simulink model "TVC_6DOF_Model_WJHedits_2024a"  (R2024b)
settings: Solver=VariableStepAuto  StartTime=0.0  StopTime=8  FixedStep=.0001  RelTol=1e-6
values from neighbouring files (symbols this model uses):
  dt = 1/400    (= 0.0025)    [quaternionLQR_WJHedits.m]
  K = lqr(A,B, Q, R)    [quaternionLQR_WJHedits.m]
  mass = .89    (= 0.89)    [quaternionLQR_WJHedits.m]
  maxGimbal = deg2rad(8)    [quaternionLQR_WJHedits.m]
  momentArm = 0.49    [quaternionLQR_WJHedits.m]
  q_init = angle2quat(euler_init(3),euler_init(2),euler_init(1),'ZYX')    [quaternionLQR_WJHedits.m]
  servoRatio = 3.3    [quaternionLQR_WJHedits.m]
  T = 15    [quaternionLQR_WJHedits.m]
  thrust = data{:,2}    [quaternionLQR_WJHedits.m]
  time = data{:,1}    [quaternionLQR_WJHedits.m]
undefined symbols (not defined in the file or in its folder): prop
libraries: simulink x4, sharedtransform x1, shared6dof x1, aerolibanim x1
settings Model: Creator=lucan  LastModifiedBy=C27Nathan.Aldridge

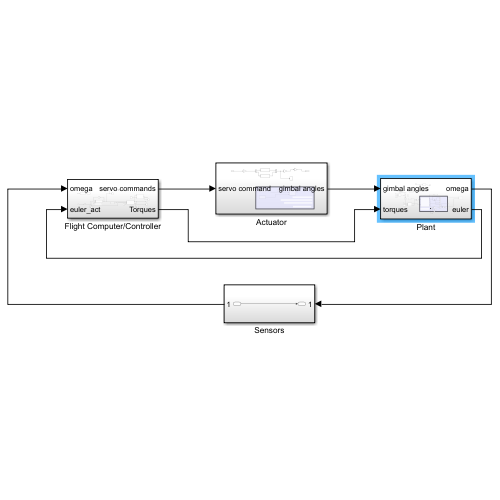
[thumbnail: Simulink's stored preview of the top-level diagram]
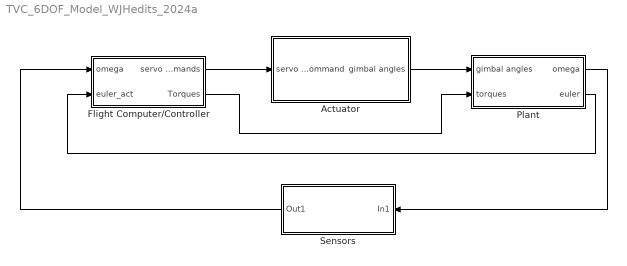
== system TVC_6DOF_Model_WJHedits_2024a ==
  Actuator : Subsystem
  Flight Computer/Controller : Subsystem
  Plant : Subsystem
  Sensors : Subsystem
  wires:
  Plant/1(omega) -> Sensors/1(In1)
  Sensors/1(Out1) -> Flight Computer/Controller/1(omega)
  Flight Computer/Controller/1(" servo commands") -> Actuator/1(servo command)
  Actuator/1(gimbal angles) -> Plant/1(gimbal angles)
  Plant/2(euler) -> Flight Computer/Controller/2(euler_act)
  Flight Computer/Controller/2(Torques) -> Plant/2(torques)

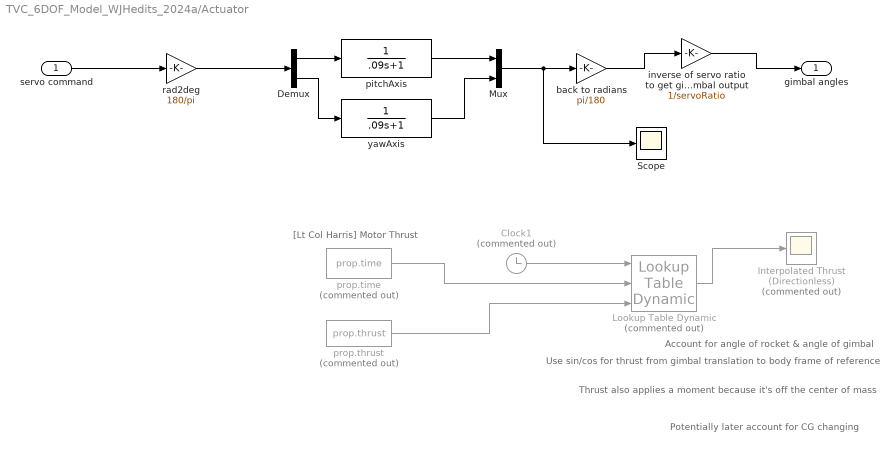
== system TVC_6DOF_Model_WJHedits_2024a/Actuator ==
  note: Potentially later account for CG changing
  note: Thrust also applies a moment because it's off the center of mass
  note: Account for angle of rocket & angle of gimbal
  note: [Lt Col Harris] Motor Thrust
  note: Use sin/cos for thrust from gimbal translation to body frame of reference
  servo command : Inport
  Clock1 : Clock  Commented=on
  Demux : Demux  Outputs=2
  Interpolated Thrust (Directionless) : Scope  Commented=on
  Lookup Table Dynamic : simulink/Lookup Tables/Lookup Table Dynamic  Commented=on  LookUpMeth=Interpolation-Use End Values  OutDataType=fixdt('double')  OutScaling=[]  OutputDataTypeScalingMode=Specify via dialog  OutDataTypeStr=double  DoSatur=off
  Mux : Mux  Inputs=2
  Scope : Scope
  back to radians : Gain  Gain=pi/180
  inverse of servo ratio to get gimbal output : Gain  Gain=1/servoRatio
  pitchAxis : TransferFcn  Denominator=[.09 1]  ContinuousStateAttributes='servoposition'
  prop.thrust : Constant  Commented=on  Value=prop.thrust
  prop.time : Constant  Commented=on  Value=prop.time
  rad2deg : Gain  Gain=180/pi
  yawAxis : TransferFcn  Denominator=[.09 1]  ContinuousStateAttributes='servoposition'
  gimbal angles : Outport
  wires:
  prop.time/1 -> Lookup Table Dynamic/2
  prop.thrust/1 -> Lookup Table Dynamic/3
  Lookup Table Dynamic/1 -> Interpolated Thrust (Directionless)/1
  Clock1/1 -> Lookup Table Dynamic/1
  servo command/1 -> rad2deg/1
  Demux/2 -> yawAxis/1
  Demux/1 -> pitchAxis/1
  pitchAxis/1 -> Mux/1
  yawAxis/1 -> Mux/2
  Mux/1 -> Scope/1, back to radians/1
  inverse of servo ratio to get gimbal output/1 -> gimbal angles/1
  rad2deg/1 -> Demux/1
  back to radians/1 -> inverse of servo ratio to get gimbal output/1

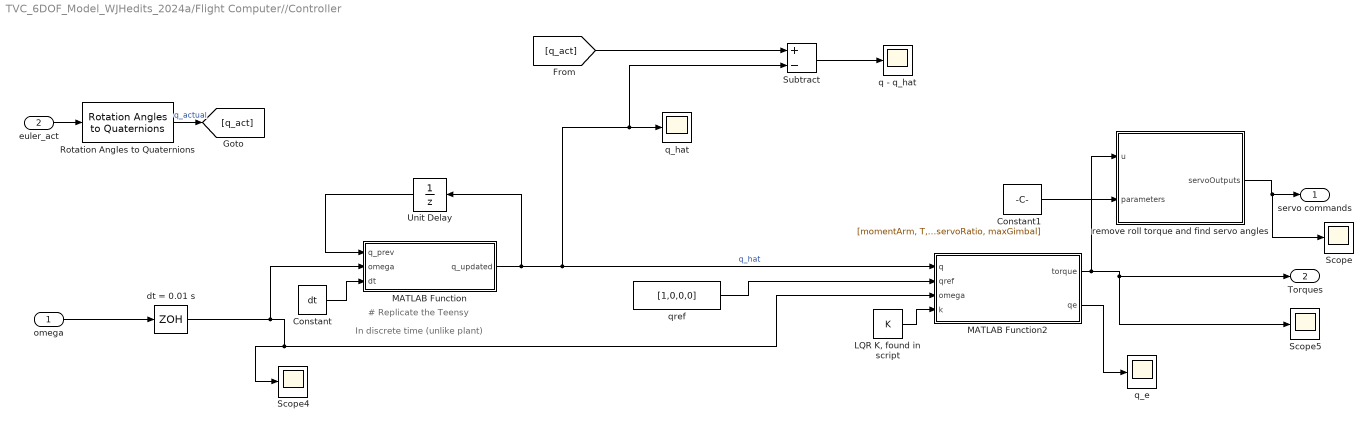
== system TVC_6DOF_Model_WJHedits_2024a/Flight Computer//Controller ==
  note: In discrete time (unlike plant)
  note: # Replicate the Teensy
  omega : Inport
  euler_act : Inport  Port=2
  Constant : Constant  Value=dt
  Constant1 : Constant  Value=[momentArm, T, servoRatio, maxGimbal]
  "LQR K, found in script" : Constant  Value=K
  MATLAB Function : MATLAB Function  TreatAsAtomicUnit=on
  MATLAB Function2 : MATLAB Function  TreatAsAtomicUnit=on
  Rotation Angles to Quaternions : sharedtransform/Rotation Angles to Quaternions  rotationOrder=XYZ  aMode=aMode
  Scope : Scope
  Scope4 : Scope
  Scope5 : Scope
  Subtract : Sum  Inputs=+-
  Unit Delay : UnitDelay  InitialCondition=q_init  SampleTime=-1  HasFrameUpgradeWarning=on
  dt = 0.01 s : ZeroOrderHold  SampleTime=dt
  q - q_hat : Scope
  q_e : Scope
  q_hat : Scope
  qref : Constant  Value=[1,0,0,0]
  remove roll torque and find servo angles : MATLAB Function  TreatAsAtomicUnit=on
  " servo commands" : Outport
  Torques : Outport  Port=2
  wires:
  Constant/1 -> MATLAB Function/3(dt)
  "LQR K, found in script"/1 -> MATLAB Function2/4(k)
  qref/1 -> MATLAB Function2/2(qref)
  MATLAB Function2/2(qe) -> q_e/1
  euler_act/1 -> Rotation Angles to Quaternions/1
  MATLAB Function/1(q_updated) -> MATLAB Function2/1(q), Subtract/2, q_hat/1, Unit Delay/1  "q_hat"
  MATLAB Function2/1(torque) -> Torques/1, Scope5/1, remove roll torque and find servo angles/1(u)
  omega/1 -> dt = 0.01 s/1
  remove roll torque and find servo angles/1(servoOutputs) -> Scope/1, " servo commands"/1
  Unit Delay/1 -> MATLAB Function/1(q_prev)
  Subtract/1 -> q - q_hat/1
  Rotation Angles to Quaternions/1 -> [q_act]  "q_actual"
  [q_act] -> Subtract/1
  dt = 0.01 s/1 -> Scope4/1, MATLAB Function2/3(omega), MATLAB Function/2(omega)
  Constant1/1 -> remove roll torque and find servo angles/2(parameters)

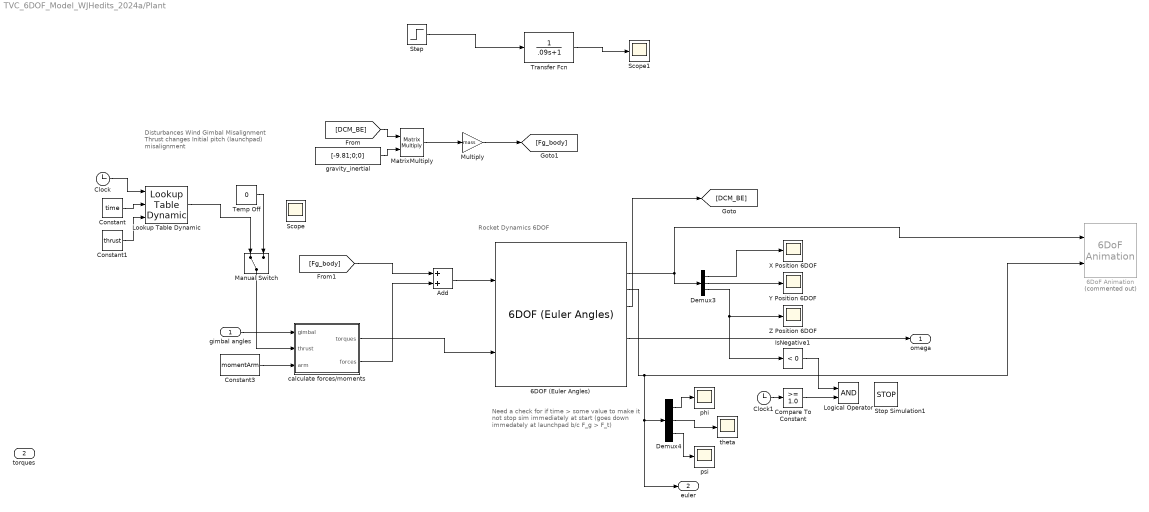
== system TVC_6DOF_Model_WJHedits_2024a/Plant ==
  note: Need a check for if time > some value to make
      | it not stop sim immediately at start (goes down
      | immedately at launchpad b/c F_g > F_t)
  note: Rocket Dynamics 6DOF
  note: Disturbances
      | Wind
      | Gimbal Misalignment
      | Thrust changes
      | Initial pitch (launchpad) misalignment
  gimbal angles : Inport
  torques : Inport  Port=2
  6DOF (Euler Angles) : shared6dof/6DOF (Euler Angles)  units=Metric (MKS)  mtype=Fixed  rep=Euler Angles  xme_0=[0 0 0]  Vm_0=[0 0 0]  eul_0=euler_init  pm_0=w0  mass_0=1.0  mass_e=0.5  mass_f=2.0  inertia=I  inertia_e=eye(3)  inertia_f=2*eye(3)  k_quat=1.0  vre_flag=on  abi_flag=off  aMode=0  xme_statename=''  Vm_statename=''  eul_statename=''  quat_statename=''  pm_statename=''  mass_statename=''
  6DoF Animation : aerolibanim/6DoF Animation  Commented=on  u1=[-10 100 -50 50 -50 50]  u2=.03  u3=20  u4=[0,1000,0]  u5=Fixed position  u6=[50,50,50]  u7=40  u8=on
  Add : Sum
  Clock : Clock
  Clock1 : Clock
  Compare To Constant : simulink/Logic and Bit Operations/Compare To Constant  relop=>=  const=1.0  OutDataTypeStr=boolean
  Constant : Constant  Value=time
  Constant1 : Constant  Value=thrust
  Constant3 : Constant  Value=momentArm
  Demux3 : Demux  Outputs=3
  Demux4 : Demux  Outputs=3
  IsNegative1 : simulink/Logic and Bit Operations/Compare To Zero  relop=<  OutDataTypeStr=boolean
  Logical Operator : Logic  AllPortsSameDT=off  OutDataTypeStr=boolean
  Lookup Table Dynamic : simulink/Lookup Tables/Lookup Table Dynamic  LookUpMeth=Interpolation-Use End Values  OutDataType=fixdt('double')  OutScaling=[]  OutputDataTypeScalingMode=Specify via dialog  OutDataTypeStr=double  DoSatur=off
  Manual Switch : ManualSwitch
  MatrixMultiply : Product  Multiplication=Matrix(*)
  Multiply : Gain  Gain=mass
  Scope : Scope
  Scope1 : Scope
  Step : Step  After=60  SampleTime=0
  Stop Simulation1 : Stop
  Temp Off : Constant  Value=0
  Transfer Fcn : TransferFcn  Denominator=[.09 1]
  X Position 6DOF : Scope
  Y Position 6DOF : Scope
  Z Position 6DOF : Scope
  calculate forces/moments : MATLAB Function  TreatAsAtomicUnit=on
  gravity_inertial : Constant  Value=[-9.81;0;0]
  phi : Scope
  psi : Scope
  theta : Scope
  omega : Outport
  euler : Outport  Port=2
  wires:
  6DOF (Euler Angles)/2 -> Demux3/1, 6DoF Animation/1
  Demux3/3 -> IsNegative1/1, Z Position 6DOF/1
  Manual Switch/1 -> calculate forces/moments/2(thrust)
  Demux3/1 -> X Position 6DOF/1
  Demux3/2 -> Y Position 6DOF/1
  Clock1/1 -> Compare To Constant/1
  Compare To Constant/1 -> Logical Operator/2
  IsNegative1/1 -> Logical Operator/1
  Temp Off/1 -> Manual Switch/2
  Demux4/1 -> phi/1
  Demux4/2 -> theta/1
  Demux4/3 -> psi/1
  6DOF (Euler Angles)/3 -> Demux4/1, euler/1, 6DoF Animation/2
  6DOF (Euler Angles)/6 -> omega/1
  6DOF (Euler Angles)/4 -> [DCM_BE]
  [DCM_BE] -> MatrixMultiply/1
  gravity_inertial/1 -> MatrixMultiply/2
  MatrixMultiply/1 -> Multiply/1
  Multiply/1 -> [Fg_body]
  gimbal angles/1 -> calculate forces/moments/1(gimbal)
  calculate forces/moments/1(torques) -> 6DOF (Euler Angles)/2
  Clock/1 -> Lookup Table Dynamic/1
  Constant/1 -> Lookup Table Dynamic/2
  Constant1/1 -> Lookup Table Dynamic/3
  Lookup Table Dynamic/1 -> Manual Switch/1
  Constant3/1 -> calculate forces/moments/3(arm)
  Add/1 -> 6DOF (Euler Angles)/1
  calculate forces/moments/2(forces) -> Add/2
  [Fg_body] -> Add/1
  Step/1 -> Transfer Fcn/1
  Transfer Fcn/1 -> Scope1/1

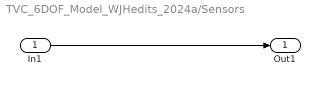
== system TVC_6DOF_Model_WJHedits_2024a/Sensors ==
  In1 : Inport
  Out1 : Outport
  wires:
  In1/1 -> Out1/1

== matlab function TVC_6DOF_Model_WJHedits_2024a/Flight Computer//Controller/remove roll torque and find servo angles ==
  data: u input; servoOutputs output; parameters input
function servoOutputs = calculateServo(u, parameters)
  %define parameters locally
  momentArm = parameters(1);
  thrust = parameters(2);
  servoRatio = parameters(3);
  maxGimbal = parameters(4);
  torque = [u(2), u(3)]; %grab torques we can actually use
  gimbal = [torque(1)/ (momentArm * thrust), torque(2)/ (momentArm * thrust)];
  for i = 1:length(gimbal)
     if abs(gimbal(i)) > maxGimbal
        gimbal(i) = maxGimbal * gimbal(i)/abs(gimbal(i));
     end
  end
  servoOutputs = gimbal*servoRatio; %in radians
end

== matlab function TVC_6DOF_Model_WJHedits_2024a/Flight Computer//Controller/MATLAB Function ==
  data: q_prev input; q_updated output; omega input; dt input
function q_updated = update_quaternion(q_prev, omega, dt)
    % q: Current quaternion [w, x, y, z]
    q_prev = [q_prev(1), q_prev(2), q_prev(3), q_prev(4)];
    % q = [q(2), q(3), q(4), q(1)];
    %ensure w is a row vector
    w = [omega(1), omega(2), omega(3),0];
    
    A = [0 -w(1) -w(2) -w(3);
        w(1) 0 w(3) -w(2);
        w(2) -w(3) 0 w(1);
        w(3) w(2) -w(1) 0];

    B = [q_prev(1) -q_prev(2) -q_prev(3) -q_prev(4);
        q_prev(2) q_prev(1) -q_prev(4) q_prev(3);
        q_prev(3) q_prev(4) q_prev(1) -q_prev(2);
        q_prev(4) -q_prev(3) q_prev(2) q_prev(1)];

    G = [q_prev(4) -q_prev(3) q_prev(2) q_prev(1);
         q_prev(3) q_prev(4) -q_prev(1) q_prev(2);
        -q_prev(2) q_prev(1) q_prev(4) q_prev(3);
        -q_prev(1) -q_prev(2) -q_prev(3) q_prev(4)];

   qdot = 0.5*A*q_prev';
   % qdot = 0.5*G*w';

   q_updated = q_prev + (qdot*dt)';

    % Normalize to prevent drift
    q_updated = q_updated / norm(q_updated);

    % q_updated = [q_updated(4), q_updated(1), q_updated(2), q_updated(3)];
end

== matlab function TVC_6DOF_Model_WJHedits_2024a/Flight Computer//Controller/MATLAB Function2 ==
  data: q input; torque output; qref input; omega input; k input; qe output
function [torque,qe] = quaternion_control_law(q, qref, omega, k)
    % Compute the conjugate of the quaternion
    q = [q(1), q(2), q(3), q(4)];
    qref_conj = [qref(1), -qref(2), -qref(3), -qref(4)];

    %compute norm
    norm_squared = qref(1)^2 + qref(2)^2 + qref(3)^2 + qref(4)^2;

    % Compute the inverse of the quaternion
    qref_inv = qref_conj / norm_squared;
    
    %find qe
    % qe = quatmultiply(qref_inv, q);
    qe = q;

    %take the last 3 elements of q as used in the state space and the omega
    I = diag([.05, .1, .1]);
    torque = -k*[[qe(2); qe(3); qe(4)]; omega] + cross(omega,I*omega);
end

== matlab function TVC_6DOF_Model_WJHedits_2024a/Plant/calculate forces//moments ==
  data: gimbal input; torques output; thrust input; forces output; arm input
function [torques, forces] = fcn(gimbal, thrust, arm)
    torques = [0, thrust * sin(gimbal(1))*arm, thrust * sin(gimbal(2))*arm];
    forces = [thrust * cos(gimbal(1)) * cos(gimbal(2)), thrust * sin(gimbal(2)), thrust * sin(gimbal(1))];
end
